simulink model "component_model"  (R2014a)
settings: Solver=ode45  StartTime=0.0  StopTime=30  RelTol=1e-3
libraries: simulink x2, CivilEnginelibV1 x1
settings Model: Creator=mmm  LastModifiedBy=mmm

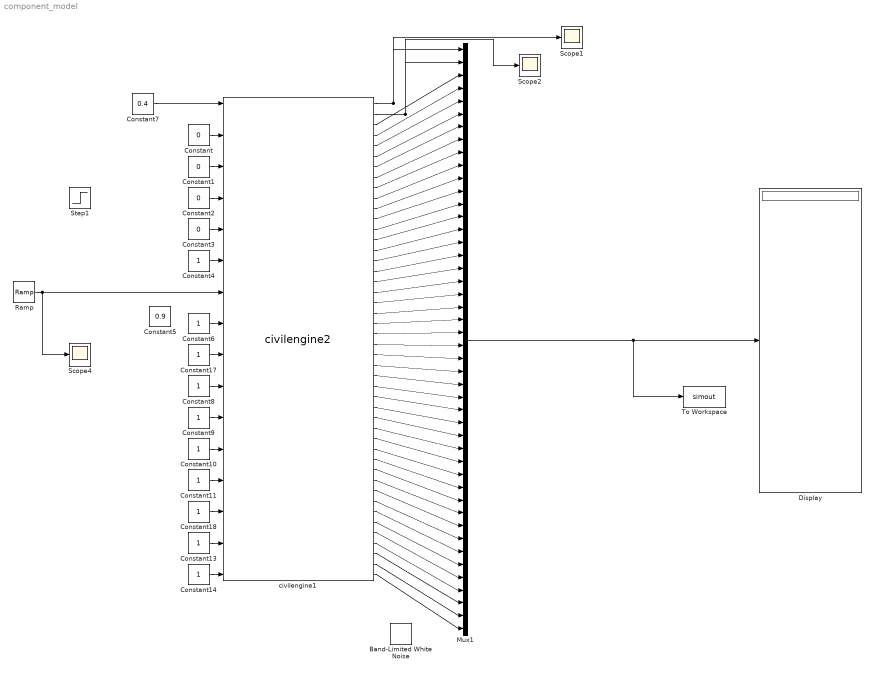
== system component_model ==
  Band-Limited White Noise : simulink/Sources/Band-Limited White Noise  Cov=[10*0.02]  Ts=0.02  seed=[23341]
  Constant{,1..3} (4 alike) : Constant  Value=0
  Constant{4,6,8..11,13..14,17..18} (10 alike) : Constant
  Constant5 : Constant  Value=0.9
  Constant7 : Constant  Value=0.4
  Display : Display
      settings: Decimation=46
  Mux1 : Mux  Inputs=46
  Ramp : simulink/Sources/Ramp  slope=-0.005  start=10  X0=1
  Scope1 : Scope
      settings: YMin=5000.04  YMax=5000.05
  Scope2 : Scope
  Scope4 : Scope
      settings: SaveName=ScopeData3
  Step1 : Step  Time=10  Before=1  After=0.9  SampleTime=0
  To Workspace : ToWorkspace  VariableName=simout  SampleTime=-1
  civilengine1 : CivilEnginelibV1/civilengine2  Ts=0.02  delta_T=0
  wires:
  Constant/1 -> civilengine1/2
  Constant1/1 -> civilengine1/3
  Constant2/1 -> civilengine1/4
  Constant3/1 -> civilengine1/5
  Constant4/1 -> civilengine1/6
  Constant6/1 -> civilengine1/8
  Constant8/1 -> civilengine1/10
  Constant9/1 -> civilengine1/11
  Constant10/1 -> civilengine1/12
  Constant11/1 -> civilengine1/13
  Constant13/1 -> civilengine1/15
  Constant14/1 -> civilengine1/16
  Constant17/1 -> civilengine1/9
  Constant18/1 -> civilengine1/14
  civilengine1/1 -> Mux1/1, Scope1/1
  civilengine1/2 -> Mux1/2, Scope2/1
  civilengine1/3 -> Mux1/3
  civilengine1/4 -> Mux1/4
  civilengine1/5 -> Mux1/5
  civilengine1/6 -> Mux1/6
  civilengine1/7 -> Mux1/7
  civilengine1/8 -> Mux1/8
  civilengine1/9 -> Mux1/9
  civilengine1/10 -> Mux1/10
  civilengine1/11 -> Mux1/11
  civilengine1/12 -> Mux1/12
  civilengine1/13 -> Mux1/13
  civilengine1/14 -> Mux1/14
  civilengine1/15 -> Mux1/15
  civilengine1/16 -> Mux1/16
  civilengine1/17 -> Mux1/17
  civilengine1/18 -> Mux1/18
  civilengine1/19 -> Mux1/19
  civilengine1/20 -> Mux1/20
  civilengine1/21 -> Mux1/21
  civilengine1/22 -> Mux1/22
  civilengine1/23 -> Mux1/23
  civilengine1/24 -> Mux1/24
  civilengine1/25 -> Mux1/25
  civilengine1/26 -> Mux1/26
  civilengine1/27 -> Mux1/27
  civilengine1/28 -> Mux1/28
  civilengine1/30 -> Mux1/30
  civilengine1/31 -> Mux1/31
  civilengine1/32 -> Mux1/32
  civilengine1/33 -> Mux1/33
  civilengine1/34 -> Mux1/34
  civilengine1/35 -> Mux1/35
  civilengine1/36 -> Mux1/36
  civilengine1/37 -> Mux1/37
  civilengine1/38 -> Mux1/38
  civilengine1/39 -> Mux1/39
  civilengine1/40 -> Mux1/40
  civilengine1/41 -> Mux1/41
  civilengine1/42 -> Mux1/42
  civilengine1/43 -> Mux1/43
  civilengine1/44 -> Mux1/44
  civilengine1/45 -> Mux1/45
  civilengine1/46 -> Mux1/46
  Mux1/1 -> Display/1, To Workspace/1
  civilengine1/29 -> Mux1/29
  Constant7/1 -> civilengine1/1
  Ramp/1 -> Scope4/1, civilengine1/7
